simulink model "xiankong02_nolinear"  (Simulink 9.0)
settings: Solver=VariableStepAuto  StartTime=0.0  StopTime=10.0  RelTol=1e-3
values from neighbouring files (symbols this model uses):
  A = [1 0;0 2]    [xiankong01.m]    (also in xiankong02.m; xiankong03.m; xiankong03v2.m; xiankong03v4.m)
  B = [1;1]    [xiankong01.m]    (also in xiankong02.m; xiankong03.m; xiankong03v2.m; xiankong03v4.m)
  C = -C    [xiankong01.m]    (also in xiankong02.m; xiankong03.m = [1 2]; xiankong03v2.m = [1 2]; xiankong03v4.m = [1 2])
  K = acker(A,B,P)    [xiankong01.m]    (also in xiankong02.m; xiankong03.m = acker(AA,BB,P); xiankong03v2.m = acker(AA,BB,P); xiankong03v4.m = acker(AA,BB,P))
  L = (acker(A',C',Q))'    [xiankong02.m]    (also in xiankong04.m; xiankong04v2.m; xiankong05.m)
  s_max = s_value    (= 10)    [xiankong01.m]    (also in xiankong02.m; xiankong03.m; xiankong03v2.m; xiankong03v4.m = 0.01)
  s_min = -s_value    (= -10)    [xiankong01.m]    (also in xiankong02.m; xiankong03.m; xiankong03v2.m; xiankong03v4.m = -0.01)
  u_k = 10    [xiankong01.m]    (also in xiankong02.m; xiankong05.m = 1)
settings Model: Creator=wulin  LastModifiedBy=wulin
settings DataIOCC: SaveFormat=Dataset
settings OptimizationCC: LifeSpan=auto
settings DebuggingCC: UnderspecifiedInitializationDetection=Simplified  MergeDetectMultiDrivingBlocksExec=error  SFUnexpectedBacktrackingDiag=error  SFNoUnconditionalDefaultTransitionDiag=error  SFExecutionAtInitializationDiag=warning
settings HardwareCC: ProdBitPerPointer=64  ProdBitPerSizeT=64  ProdBitPerPtrDiffT=64  ProdLargestAtomicFloat=Float  ProdIntDivRoundTo=Zero  ProdEndianess=LittleEndian  ProdWordSize=64  ProdHWDeviceType=Intel->x86-64 (Windows64)
settings ModelReferenceCC: PropagateSignalLabelsOutOfModel=on
settings CodeAppCC: StateflowObjectComments=off
settings GRTTargetCC: TargetLangStandard=C99 (ISO)
settings ConfigComp: CovMetricSettings=dwe  CovHtmlReporting=off  CovSaveCumulativeToWorkspaceVar=off  CovSaveSingleToWorkspaceVar=off  CovExternalEMLEnable=on

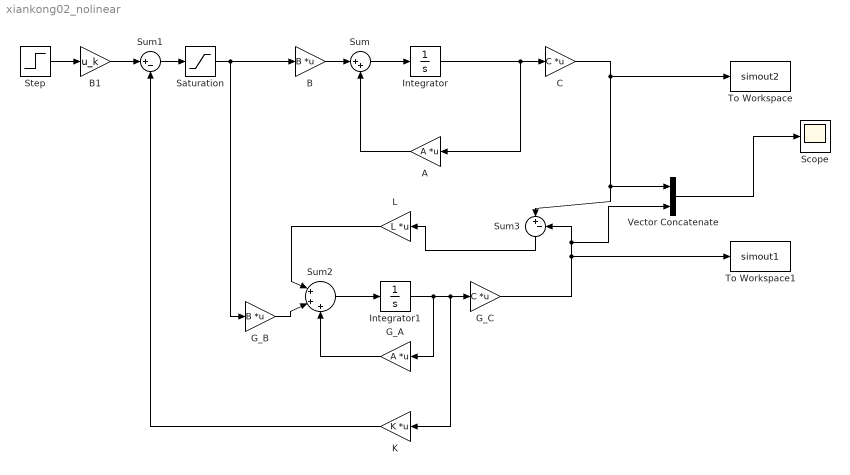
== system xiankong02_nolinear ==
  "A " : Gain  Gain=A  Multiplication=Matrix(K*u) (u vector)
  B : Gain  Gain=B  Multiplication=Matrix(K*u) (u vector)
  B1 : Gain  Gain=u_k
  C : Gain  Gain=C  Multiplication=Matrix(K*u) (u vector)
  G_A : Gain  Gain=A  Multiplication=Matrix(K*u) (u vector)
  G_B : Gain  Gain=B  Multiplication=Matrix(K*u) (u vector)
  "G_C " : Gain  Gain=C  Multiplication=Matrix(K*u) (u vector)
  Integrator : Integrator
  Integrator1 : Integrator
  "K " : Gain  Gain=K  Multiplication=Matrix(K*u) (u vector)
  L : Gain  Gain=L  Multiplication=Matrix(K*u) (u vector)
  Saturation : Saturate  UpperLimit=s_max  LowerLimit=s_min
  Scope : Scope
  Step : Step  SampleTime=0
  Sum : Sum  Inputs=|++
  Sum1 : Sum  Inputs=|+-
  Sum2 : Sum  Inputs=|+++
  Sum3 : Sum  Inputs=|+-
  To Workspace : ToWorkspace  VariableName=simout2  SampleTime=-1
  To Workspace1 : ToWorkspace  VariableName=simout1  SampleTime=-1
  Vector Concatenate : Concatenate
  wires:
  Integrator/1 -> C/1, "A "/1
  B/1 -> Sum/1
  "A "/1 -> Sum/2
  Sum/1 -> Integrator/1
  Sum1/1 -> Saturation/1
  Saturation/1 -> B/1, G_B/1
  B1/1 -> Sum1/1
  Step/1 -> B1/1
  Integrator1/1 -> G_A/1, "K "/1, "G_C "/1
  G_A/1 -> Sum2/3
  G_B/1 -> Sum2/2
  Sum3/1 -> L/1
  L/1 -> Sum2/1
  "G_C "/1 -> To Workspace1/1, Vector Concatenate/2, Sum3/2
  Sum2/1 -> Integrator1/1
  "K "/1 -> Sum1/2
  Vector Concatenate/1 -> Scope/1
  C/1 -> To Workspace/1, Vector Concatenate/1, Sum3/1
